simulink model "agg_all_simulated_unitIDs_example"  (R2015a)
settings: Solver=FixedStepDiscrete  StartTime=0.0  StopTime=inf  FixedStep=60  RelTol=1e-3
libraries: libAggregators x2, libSimulators x2
settings Model: Creator=jcardena  LastModifiedBy=BCao

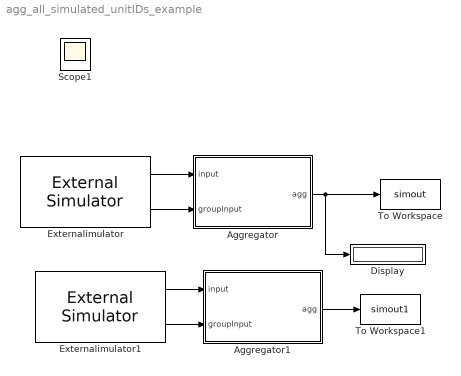
== system agg_all_simulated_unitIDs_example ==
  Aggregator : Subsystem  BlockChoice=Simplest
      settings: AttributesFormatString=%<BlockChoice>  TemplateBlock=libAggregators/Aggregator  MemberBlocks=Average,Simple,Simple db Aggregator,Simplest
  Aggregator1 : Subsystem  BlockChoice=Simplest
      settings: AttributesFormatString=%<BlockChoice>  TemplateBlock=libAggregators/Aggregator  MemberBlocks=Average,Simple,Simple db Aggregator,Simplest
  Display : Display
  Externalimulator : libSimulators/External Simulator  Condition=%20151221%  N=100  db_name=HeatingUnits  db_username=sw_ETS  db_password=unb.sql.2015
  Externalimulator1 : libSimulators/External Simulator  Condition=%20151222%  N=200  db_name=WaterHeaters  db_username=sw_waterheaters  db_password=unb.sql.2015
  To Workspace : ToWorkspace  VariableName=simout  SaveFormat=Structure With Time  SampleTime=-1
  To Workspace1 : ToWorkspace  VariableName=simout1  SaveFormat=Structure With Time  SampleTime=-1
  Scope1 : Scope
  wires:
  Externalimulator/2 -> Aggregator/2(groupInput)
  Externalimulator/1 -> Aggregator/1(input)
  Aggregator/1(agg) -> Display/1, To Workspace/1
  Aggregator1/1(agg) -> To Workspace1/1
  Externalimulator1/1 -> Aggregator1/1(input)
  Externalimulator1/2 -> Aggregator1/2(groupInput)

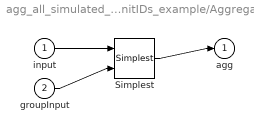
== system agg_all_simulated_unitIDs_example/Aggregator ==
  input : Inport
  groupInput : Inport  Port=2
  Simplest : libAggregators/Simplest  SystemSampleTime=-1
  agg : Outport
  wires:
  input/1 -> Simplest/1
  groupInput/1 -> Simplest/2
  Simplest/1 -> agg/1

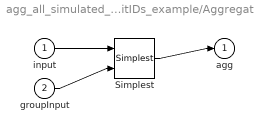
== system agg_all_simulated_unitIDs_example/Aggregator1 ==
  input : Inport
  groupInput : Inport  Port=2
  Simplest : libAggregators/Simplest  SystemSampleTime=-1
  agg : Outport
  wires:
  input/1 -> Simplest/1
  groupInput/1 -> Simplest/2
  Simplest/1 -> agg/1
